simulink model "lab3_3"  (R2020b)
settings: Solver=VariableStepAuto  StartTime=0.0  StopTime=300  MaxStep=0.01  RelTol=1e-3
InitFcn:
  | a0 = 2;
  | a1 = -5;
  | b0 = 5;
  | A = [0 1; -a0 -a1];
  | b = [0; b0];
  | 
  | am0 = 64;
  | am1 = 16;
  | Am = [0 1; -am0 -am1];
  | bm = [0; am0];
  | 
  | theta1 = (a0 - am0)/b0;
  | theta2 = (a1 - am1)/b0;
  | kappa = b0/am0;
  | 
  | Q = eye(2);
  | P = lyap(Am', Q);
undefined symbols (not defined in the file): theta
settings Model: Creator=Eeer12  LastModifiedBy=Eugene

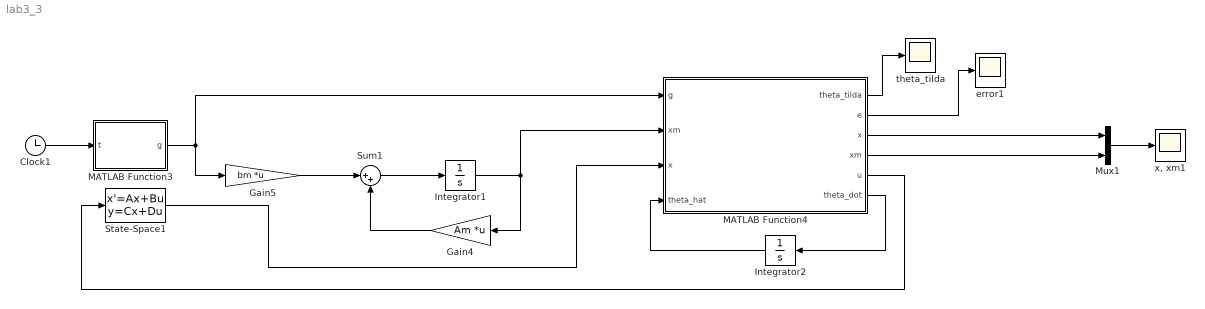
== system lab3_3 ==
  Clock1 : Clock
  Gain4 : Gain  Gain=Am  Multiplication=Matrix(K*u)
  Gain5 : Gain  Gain=bm  Multiplication=Matrix(K*u)
  Integrator1 : Integrator  InitialCondition=[0; 0]
  Integrator2 : Integrator  InitialCondition=[0; 0]
  MATLAB Function3 : MATLAB Function  TreatAsAtomicUnit=on
  MATLAB Function4 : MATLAB Function  TreatAsAtomicUnit=on
  Mux1 : Mux  Inputs=2
  State-Space1 : StateSpace  A=A + [0 0; 20 20]  B=b  C=eye(2)  D=[0; 0]  InitialCondition=[0; 0]
  Sum1 : Sum  Inputs=|++
  error1 : Scope
  theta_tilda : Scope
  "x, xm1" : Scope
  wires:
  MATLAB Function3/1(g) -> Gain5/1, MATLAB Function4/1(g)
  State-Space1/1 -> MATLAB Function4/3("x ")
  Sum1/1 -> Integrator1/1
  Clock1/1 -> MATLAB Function3/1(t)
  Integrator1/1 -> Gain4/1, MATLAB Function4/2("xm ")
  MATLAB Function4/3(x) -> Mux1/1
  MATLAB Function4/2(e) -> error1/1
  Gain4/1 -> Sum1/2
  MATLAB Function4/4(xm) -> Mux1/2
  MATLAB Function4/5(u) -> State-Space1/1
  Gain5/1 -> Sum1/1
  Mux1/1 -> "x, xm1"/1
  MATLAB Function4/6(theta_dot) -> Integrator2/1
  Integrator2/1 -> MATLAB Function4/4(theta_hat)
  MATLAB Function4/1(theta_tilda) -> theta_tilda/1

== matlab function lab3_3/MATLAB Function3 ==
  data: t input; g output
function g = fcn(t)

g = 10*cos(0.5*t) + 2*sin(t) + 12;

== matlab function lab3_3/MATLAB Function4 ==
  data: theta_tilda output; e output; x output; xm output; g input; xm input; x input; u output; kappa parameter; theta parameter; theta_hat input; theta_dot output; P parameter; b parameter
function [theta_tilda, e, x, xm, u, theta_dot] = fcn(g, xm, x, kappa, theta, theta_hat, P, b)

gamma = 100;
e = xm-x;
theta_dot = gamma*x*b'*P*e;
u = theta_hat'*x + g/kappa;
theta_tilda = theta - theta_hat;
